simulink library "tethersNCsContrl_cl"  (R2018b)
settings: Solver=VariableStepAuto  StartTime=0.0  StopTime=10.0  RelTol=1e-3
undefined symbols (not defined in the file or in its folder): ctrllr
libraries: filteredPIDController_ul x5
settings Model: Creator=Ayaz  LastModifiedBy=asiddiq2

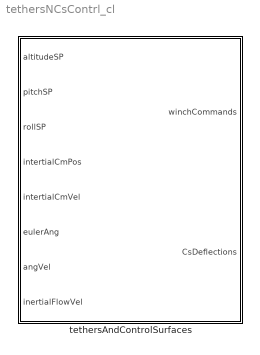
== system tethersNCsContrl_cl ==
  tethersAndControlSurfaces : Subsystem  mask{thr_clr=ctrllr.tethers, cs_clr=ctrllr.controlSurfaces}
      mask prompts: thr_clr "Tether Controller"; cs_clr "CS controller"

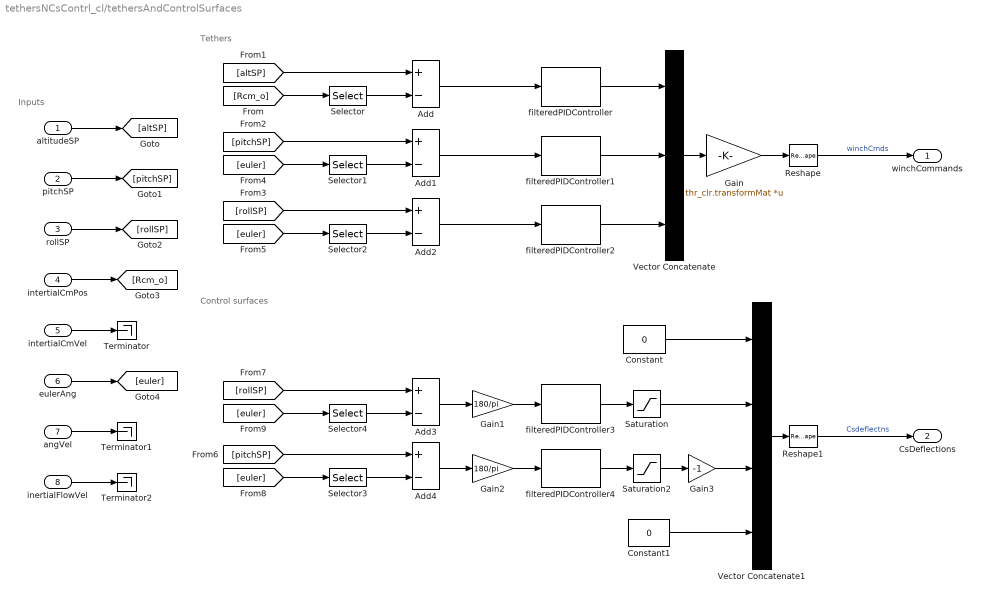
== system tethersNCsContrl_cl/tethersAndControlSurfaces ==
  note: Inputs
  note: Control surfaces
  note: Tethers
  altitudeSP : Inport
  pitchSP : Inport  Port=2
  rollSP : Inport  Port=3
  intertialCmPos : Inport  Port=4
  intertialCmVel : Inport  Port=5
  eulerAng : Inport  Port=6
  angVel : Inport  Port=7
  inertialFlowVel : Inport  Port=8
  Add{,1..4} (5 alike) : Sum  Inputs=+-
  Constant : Constant  Value=0
  Constant1 : Constant  Value=0
  Gain : Gain  Gain=thr_clr.transformMat  Multiplication=Matrix(K*u)
  Gain1 : Gain  Gain=180/pi
  Gain2 : Gain  Gain=180/pi
  Gain3 : Gain  Gain=-1
  Reshape : Reshape  OutputDimensionality=Row vector (2-D)
  Reshape1 : Reshape  OutputDimensionality=Column vector (2-D)
  Saturation : Saturate  UpperLimit=cs_clr.aileronMaxDef  LowerLimit=-cs_clr.aileronMaxDef
  Saturation2 : Saturate  UpperLimit=cs_clr.elevatorMaxDef  LowerLimit=-cs_clr.elevatorMaxDef
  Selector : Selector  NumberOfDimensions=2  InputPortWidth=3  IndexOptions=Index vector (dialog),Index vector (dialog)  Indices=3,1  OutputSizes=1,1
  Selector1 : Selector  NumberOfDimensions=2  InputPortWidth=3  IndexOptions=Index vector (dialog),Index vector (dialog)  Indices=2,1  OutputSizes=1,1
  Selector2 : Selector  NumberOfDimensions=2  InputPortWidth=3  IndexOptions=Index vector (dialog),Index vector (dialog)  Indices=1,1  OutputSizes=1,1
  Selector3 : Selector  NumberOfDimensions=2  InputPortWidth=3  IndexOptions=Index vector (dialog),Index vector (dialog)  Indices=2,1  OutputSizes=1,1
  Selector4 : Selector  NumberOfDimensions=2  InputPortWidth=3  IndexOptions=Index vector (dialog),Index vector (dialog)  Indices=1,1  OutputSizes=1,1
  Terminator : Terminator
  Terminator1 : Terminator
  Terminator2 : Terminator
  Vector Concatenate : Concatenate  NumInputs=3
  Vector Concatenate1 : Concatenate  NumInputs=4
  filteredPIDController : filteredPIDController_ul/filteredPIDController  kp=thr_clr.altiTetherKp  ki=thr_clr.altiTetherKi  kd=thr_clr.altiTetherKd  Value=thr_clr.altiTetherTau
  filteredPIDController1 : filteredPIDController_ul/filteredPIDController  kp=thr_clr.pitchTetherKp  ki=thr_clr.pitchTetherKi  kd=thr_clr.pitchTetherKd  Value=thr_clr.pitchTetherTau
  filteredPIDController2 : filteredPIDController_ul/filteredPIDController  kp=thr_clr.rollTetherKp  ki=thr_clr.rollTetherKi  kd=thr_clr.rollTetherKd  Value=thr_clr.rollTetherTau
  filteredPIDController3 : filteredPIDController_ul/filteredPIDController  kp=cs_clr.aileronKp  ki=cs_clr.aileronKi  kd=cs_clr.aileronKd  Value=cs_clr.aileronTau
  filteredPIDController4 : filteredPIDController_ul/filteredPIDController  kp=cs_clr.elevatorKp  ki=cs_clr.elevatorKi  kd=cs_clr.elevatorKd  Value=cs_clr.elevatorTau
  winchCommands : Outport
  CsDeflections : Outport  Port=2
  wires:
  [altSP] -> Add/1
  [Rcm_o] -> Selector/1
  Selector/1 -> Add/2
  Selector1/1 -> Add1/2
  [pitchSP] -> Add1/1
  Selector2/1 -> Add2/2
  [rollSP] -> Add2/1
  [euler] -> Selector1/1
  [euler] -> Selector2/1
  Add2/1 -> filteredPIDController2/1
  Add1/1 -> filteredPIDController1/1
  Add/1 -> filteredPIDController/1
  filteredPIDController1/1 -> Vector Concatenate/2
  filteredPIDController/1 -> Vector Concatenate/1
  filteredPIDController2/1 -> Vector Concatenate/3
  Vector Concatenate/1 -> Gain/1
  Add3/1 -> Gain1/1
  Add4/1 -> Gain2/1
  filteredPIDController3/1 -> Saturation/1
  filteredPIDController4/1 -> Saturation2/1
  Selector3/1 -> Add4/2
  [euler] -> Selector3/1
  [pitchSP] -> Add4/1
  Selector4/1 -> Add3/2
  [rollSP] -> Add3/1
  [euler] -> Selector4/1
  Constant/1 -> Vector Concatenate1/1
  Saturation/1 -> Vector Concatenate1/2
  Saturation2/1 -> Gain3/1
  Constant1/1 -> Vector Concatenate1/4
  Vector Concatenate1/1 -> Reshape1/1
  altitudeSP/1 -> [altSP]
  pitchSP/1 -> [pitchSP]
  rollSP/1 -> [rollSP]
  intertialCmPos/1 -> [Rcm_o]
  eulerAng/1 -> [euler]
  intertialCmVel/1 -> Terminator/1
  angVel/1 -> Terminator1/1
  inertialFlowVel/1 -> Terminator2/1
  Gain/1 -> Reshape/1
  Reshape/1 -> winchCommands/1  "winchCmds"
  Reshape1/1 -> CsDeflections/1  "Csdeflectns"
  Gain1/1 -> filteredPIDController3/1
  Gain2/1 -> filteredPIDController4/1
  Gain3/1 -> Vector Concatenate1/3
